simulink library "Regler"  (R2021a)
settings: Solver=ode45  StartTime=0.0  StopTime=10.0  RelTol=1e-3
undefined symbols (not defined in the file or in its folder): k, sfunyst, sync
libraries: $bdroot x3, simulink x1
settings Model: Creator=WL  LastModifiedBy=wll
settings SolverCC: AlgebraicLoopSolver=TrustRegion
settings DataIOCC: LimitDataPoints=on  SaveFormat=Array  SignalLoggingSaveFormat=ModelDataLogs  ReturnWorkspaceOutputs=off
settings OptimizationCC: BooleanDataType=off  ExpressionDepthLimit=2147483647  InitFltsAndDblsToZero=on  LifeSpan=inf
settings DebuggingCC: SaveWithParameterizedLinksMsg=none  UnderspecifiedInitializationDetection=Classic  MergeDetectMultiDrivingBlocksExec=none  SignalResolutionControl=TryResolveAllWithWarning  MultiTaskDSMMsg=warning  MultiTaskCondExecSysMsg=none  FcnCallInpInsideContextMsg=warning  AllowSymbolicDim=off  StateNameClashWarn=warning  SFUnexpectedBacktrackingDiag=warning  SFNoUnconditionalDefaultTransitionDiag=warning  SFExecutionAtInitializationDiag=none  ArithmeticOperatorsInVariantConditions=warning
settings HardwareCC: ProdBitPerPointer=32  ProdBitPerSizeT=32  ProdBitPerPtrDiffT=32  ProdLargestAtomicFloat=None  ProdIntDivRoundTo=Undefined  ProdEndianess=Unspecified  ProdWordSize=32  ProdHWDeviceType=32-bit Generic  TargetUnknown=on
settings ModelReferenceCC: PropagateSignalLabelsOutOfModel=off
settings SFSimCC: SimUseLocalCustomCode=off  CustomCodeUndefinedFunction=UseInterfaceOnly
settings RTWCC: RTWUseLocalCustomCode=off
settings CodeAppCC: StateflowObjectComments=on
settings GRTTargetCC: TargetFcnLib=ansi_tfl_tmw.mat  TargetLangStandard=C89/C90 (ANSI)  CombineOutputUpdateFcns=off  GRTInterface=on
settings ConfigComp: CovMetricSettings=dw  CovSaveCumulativeToWorkspaceVar=on  CovSaveSingleToWorkspaceVar=on  CovExternalEMLEnable=off

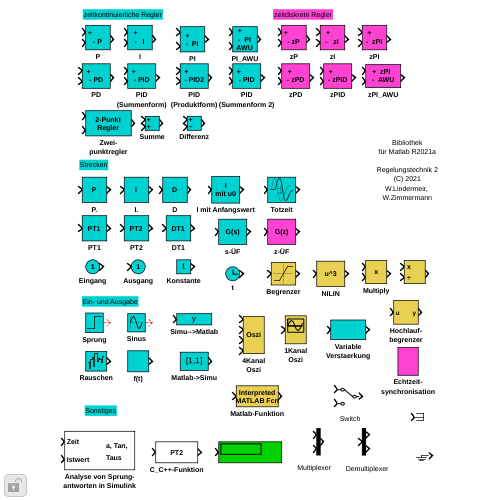
[thumbnail: Simulink's stored preview of the top-level diagram]
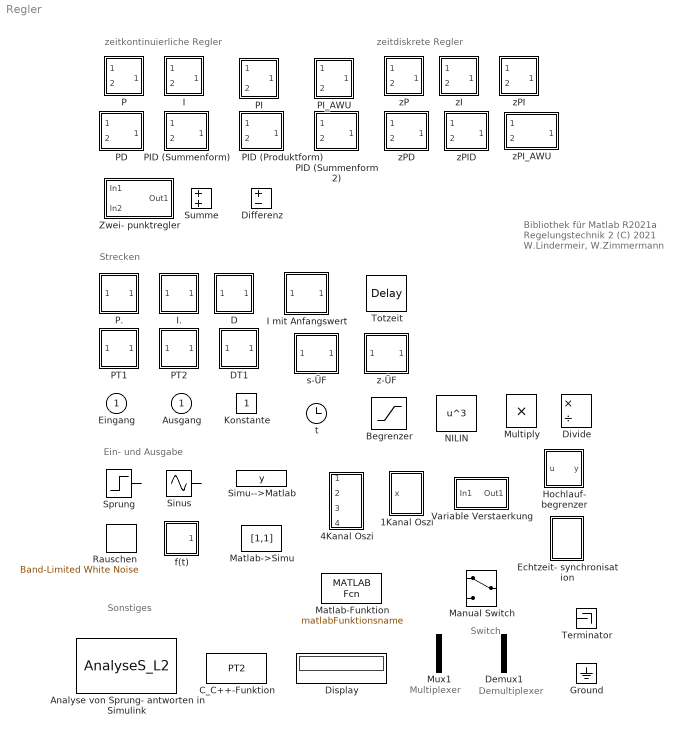
== system Regler ==
  note: Switch
  note: Ein- und Ausgabe
  note: Strecken
  note: zeitdiskrete Regler
  note: zeitkontinuierliche Regler
  note: Bibliothek
      | für Matlab R2021a
      |
      | Regelungstechnik 2
      | (C) 2021
      | W.Lindermeir,
      | W.Zimmermann
  note: Demultiplexer
  note: Multiplexer
  note: Sonstiges
  Eingang : Inport
  1Kanal Oszi : Subsystem  mask(Storage scope.){TR=1, ymin=0, ymax=1, npts=inf, color='r-/b-/g-/m-'}
      mask prompts: TR "Initial Time Range:"; ymin "Initial y-min:"; ymax "Initial y-max:"; npts "Storage pts.:"; color "Line type (rgbw-.:xo):"
      mask help:
      | Storage scope using MATLAB graph window.
      | Enter plotting ranges and line type.
      mask init:
      | ax = [0, TR, ymin, ymax]; dt=-1;
      mask Help: This block uses a MATLAB figure window to plot the input signal.  The graph limits are automatically scaled to the min and max values of the signal stored in the scope's signal buffer.  Line type must be in quotes.  See the M-file sfunyst.m.
      mask Display: plot(0,0,100,100,[83,76,63,52,42,38,28,16,11,84,11,11,11,90,90,11],[75,58,47,54,72,80,84,74,65,65,65,90,40,40,90,90])
  4Kanal Oszi : Subsystem  mask(Oszilloskop){N=20000, k=[1 1 1 1], y=[-5 5], tmax=1}
      mask prompts: N "maximale Anzahl der Abtastpunkte N:"; k "Kanalverstaerkungen:"; y "[ymin ymax]:"
      mask help:
      | 4 Kanal Oszilloskop
      | Kanal1:rot    Kanal2:blau
      | Kanal3:grün Kanal4:magenta
      |
      | Achtung: Wenn das 4 Kanal Oszilloskop mehrfach in einem Blockschaltbild
      | verwendet  wird, müssen die Bezeichnungen der Variablen x1, ..., x4 und t in
      | den Simulink->Matlab Blöcken geändert werden (Edit - Look under Mask),
      | sonst überschreiben die Signale eines Oszilloskops die Werte des anderen
      | Oszilloskops im Matlab-Workspace.
      mask Help: 4 Kanal Oszilloskop mit automat. Skalierung\nKanalverstärkung einstellbar\nKanal1:rot, Kanal2:blau\nKanal3:grün, Kanal4:magenta
      mask Display: disp('Oszi')
  Analyse von Sprung- antworten in Simulink : M-S-Function  FunctionName=AnalyseS_L2  Parameters=tol  mask(Analyse von Sprungantworten){tol=5}
      mask prompts: tol "Toleranzbereich (in %), z.B. +/-5% --> Eingabe 5"
      mask help:
      | Berechnung der Überschwingweite a, der Anregelzeit Tan und der Ausregelzeit Taus.
      |
      | Der Blockeingang ist an den Ausgang der Regelstrecke anzuschliessen.
      |
      | Die Sprungantwort muss am Ende des Zeitbereich eingeschwungen sein. Der Sprung sollte am Anfang des Zeitbereichs erfolgen.
      mask Display:
      | port_label('input',1,'Zeit');
      | port_label('input',2,'Istwert');
      | text(.6,.65,'a, Tan,');
      | text(0.6,.35,'Taus');
  Begrenzer : Saturate
  C_C++-Funktion : S-Function  FunctionName=PT2  Parameters=T  SFunctionDeploymentMode=off  EnableBusSupport=off
  D : Subsystem  mask(D){Td=1}
      mask prompts: Td "Differentiationszeitkonstante Td"
      mask help: D-Glied sTd
      mask Help: D-Glied mit Differentiationszeitkonstante Td
      mask Display: disp('D')
  DT1 : Subsystem  mask(DT1-Glied){Td=5, T1=1}
      mask help: DT1-Glied sTd/(1+sT1)
      mask Help: DT1-Glied
      mask Display: disp('DT1')
  Demux1 : Demux  Outputs=2
  Differenz : Sum  Inputs=+-  InputSameDT=on  SaturateOnIntegerOverflow=on  OutDataTypeStr=Inherit: Same as first input
  Display : Display
  Divide : Product  Inputs=*/
  Echtzeit- synchronisation : Subsystem  mask(Synchronisationsblock){T=0.1}
      mask prompts: T "Synchronistaionsperiode (min. 10ms)"
      mask help:
      | Dieser Block synchronisiert die Simulationszeit mit der realen Zeit, d.h. die Simulation läuft genauso schnell wie die reale Zeit.
      | Die Synchronisation funktioniert nur, wenn der Simulator schneller simuliert als es der realen Zeit entspricht. Der Simulator wird dann jeweils so lange angehalten, bis die reale Zeit wieder "aufgeholt" hat. Der zeitliche Abstand der Wartephasen wird durch den Parameter Synchronisationsperiode T vorgegeben. Falls dieser Block in einem Modell mit zeitdiskreten Blöcken eingesetzt wird, sollte die Synchronisationsperiode auf die (kleinste) Abtastzeit des Modells gesetzt werden. Die Synchronisationsperiode muss >= 10ms sein.
  Ground : Ground
  Hochlauf- begrenzer : Subsystem  mask(Hochlaufbegrenzer){dudt=5}
      mask prompts: dudt "Max. Änderungsgeschwindigkeit (Einheit 1/sec):"
      mask help:
      | Das Ausgangssignal folgt dem zeitlichen Verlauf des Eingangssignals exakt,
      | solange sich das Eingangssignal nicht schneller ändert als +/- du/dt. Wenn
      | sich das Eingangssignal schneller ändert, wird die Änderungsgeschwindigkeit
      | begrenzt.
  I : Subsystem  mask(I){Ti=1}
      mask prompts: Ti "Integrationszeitkonstante Ti"
      mask help: I-Glied 1/sTi
      mask Help: I-Glied mit Integrationszeitkonstante Ti
      mask Display: disp('+    \n-   I')
  I mit Anfangswert : Subsystem  mask(I-Glied 1/sTi mit Anfangswert u0){Ti=1100, u0=60}
      mask prompts: Ti "Integrationszeitkonstante Ti"; u0 "Anfangswert"
      mask help: I-Glied mit Anfangswert u0
      mask Help: Integralglied mit Anfangswert zum Zeitpunkt 0
      mask Display: disp('I\nmit u0')
  I. : Subsystem  mask(I){Ti=1}
      mask prompts: Ti "Integrationszeitkonstante Ti"
      mask help: I-Glied 1/sTi
      mask Help: I-Glied mit Integrationszeitkonstante Ti
      mask Display: disp('I')
  Konstante : Constant
  Manual Switch : ManualSwitch
  Matlab->Simu : FromWorkspace  VariableName=[1,1]  SampleTime=-1  ZeroCross=off
  Matlab-Funktion : MATLABFcn  MATLABFcn=matlabFunktionsname  OutputDimensions=3  Output1D=off
  Multiply : Product  Inputs=**
  Mux1 : Mux  Inputs=2
  NILIN : Fcn  Expr=u^3
  P : Subsystem  mask(P-Regler){kp=1}
      mask help: P
      mask Help: P-Regler mit Proportionalfaktor kp
      mask Display: disp('+        \n- P')
  P. : Subsystem  mask(P){k=1}
      mask prompts: k "Verstärkung k"
      mask help: P-Glied k
      mask Help: P-Glied mit Verstärkung k
      mask Display: disp('P')
  PD : Subsystem  mask(PD-Regler){kp=1, Tv=1, T1=0}
      mask help: PD(T1) kp (1+sTv) / (1+sT1)
      mask Help:
      | PD-Regler mit Proportionalfaktor kp und Differentiationszeitkonstante Tv.
      | Der D-Anteil wird durch ein DT1-Glied mit der zusätzlichen Tiefpasszeitkonstante T1 angenähert, es muss sein T1 >= Tv/100.
      mask Display: disp('+        \n- PD')
  PI : Subsystem  mask(PI){kp=1, Tn=1}
      mask help: PI-Regler kp (1+1/sTn)
      mask Help: PI-Regler mit Verstärkung kp und Nachstellzeit Tn
      mask Display: disp('+     \n-  PI')
  PID (Produktform) : Subsystem  mask(PID-Regler in Produktform){kr=1, Ti=1, Td=0.1, T1=0}
      mask prompts: T1 "T1  -- Achtung: Intern T1 = max(Td/100,T1)"
      mask help: PID(T1) in Produktform kr (1+sTi) (1+sTd) / sTi (1+sT1)
      mask Help:
      | PID-Regler in Produktform mit Proportionalfaktor kr, Integrationszeitkonstante Ti und Differentiationszeitkonstante Td.
      | Der D-Anteil wird durch ein DT1-Glied mit der zusätzlichen Tiefpasszeitkonstante T1 angenähert, es muss sein T1 >= Td/100.
      mask Display: disp('+        \n- PID2')
  PID (Summenform 2) : Subsystem  mask(PID-Regler in Summenform){kp=1, ki=0, kv=0, T1=0}
      mask help: PID(T1) in alternativer Summenform kp + ki/s + skv/(1+sT1) )
      mask Help:
      | PID-Regler in Summenform mit Proportionalverstärkung kp, Integralverstärkung ki und Differentialverstärkung kv.
      | Der D-Anteil wird durch ein DT1-Glied mit der zusätzlichen Tiefpasszeitkonstante T1 angenähert.
      mask Display: disp('+        \n- PID')
  PID (Summenform) : Subsystem  mask(PID-Regler in Summenform){kp=1, Tn=1, Tv=0.1, T1=0}
      mask prompts: T1 "T1  -- Achtung: Intern T1 = max(Tv/100,T1)"
      mask help: PID(T1) in Summenform kp ( 1+ 1/sTn + sTv/(1+sT1) )
      mask Help:
      | PID-Regler in Summenform mit Proportionalfaktor kp, Integrationszeitkonstante Tn (Nachstellzeit) und Differentiationszeitkonstante Tv (Vorhaltezeit).
      | Der D-Anteil wird durch ein DT1-Glied mit der zusätzlichen Tiefpasszeitkonstante T1 angenähert, es muss sein T1 >= Tv/100.
      mask Display: disp('+        \n- PID')
  PI_AWU : Subsystem  AncestorBlock=Regler/PI  mask(PI-Regler mit Anti-Windup){kp=1, Tn=0.01, bo=inf, bu=-inf}
      mask prompts: bo "Obere Begrenzung:"; bu "Untere Begrenzung:"
      mask help: PI mit Anti-Windup kp (1+sTn) / sTn
      mask Help: PI-Regler mit Proportionalfaktor kP und Integrationszeitkonstante Tn. Das Ausgangssignal wird auf den Bereich bu ... bo begrenzt. Das Einschwingverhalten bei Begrenzung wird durch eine Anti-Windup-Massnahme verbessert.
      mask Display: disp('+     \n-  PI\nAWU')
  PT1 : Subsystem  mask(PT1){k=1, T1=1}
      mask prompts: k "Verstärkung kp"; T1 "Zeitkonstante T1"
      mask help: PT1-Glied kp/(1+s·T1)
      mask Help: PT1 Tiefpaß 1.Ordnung mit Verstärkung kp und Zeitkonstante T1
      mask Display: disp('PT1')
  PT2 : Subsystem  mask(PT2){k=1, T=1, D=1}
      mask prompts: k "Verstärkung kp"; T "Zeitkonstante T1"; D "Dämpfung D"
      mask help: PT2-Glied kp/(1+s·2D·T1+s²T1²)
      mask Help: PT2 Tiefpaß 2.Ordnung mit Verstärkung kp, Zeitkonstante T1 und Daempfung D
      mask Display: disp('PT2')
  Rauschen : simulink/Sources/Band-Limited White Noise  Cov=[0.1]  Ts=0.1  seed=[23341]
  Simu-->Matlab : ToWorkspace  VariableName=y
      settings: MaxDataPoints=10000
  Sinus : Sin
  Sprung : Step  Time=0.000001  SampleTime=0
  Summe : Sum  InputSameDT=on  SaturateOnIntegerOverflow=on  OutDataTypeStr=Inherit: Same as first input
  Terminator : Terminator
  Totzeit : TransportDelay
  Variable Verstaerkung : Subsystem  LoadFcn=slideg Load  mask{Parameter4=40, k=k, Parameter5=160}
      mask prompts: Parameter4 "Low"; k "Gain"; Parameter5 "High"
      settings: CopyFcn=slideg Copy  DeleteFcn=slideg DeleteBlock  NameChangeFcn=slideg NameChange  OpenFcn=slideg Open  ParentCloseFcn=slideg ParentClose
      mask Display: disp(k)
  Zwei- punktregler : Subsystem  mask(Zweipunktregler){Yo=1, Yu=-1, So=0.1, Su=-0.1}
      mask prompts: Yo "Ausgangsignal oberer Wert:"; Yu "Ausgangssignal unterer Wert:"; So "Schaltschwelle oberer Wert:"; Su "Schaltschwelle unterer Wert:"
      mask help: Zweipunktregler mit Hysterese
      mask Help: Zweipunktregler mit Hysterese
      mask Display: fprintf('2-Punkt\nRegler')
  f(t) : Subsystem
  s-ÜF : Subsystem  mask(G(s)){Z=[0 1], N=[1 1]}
      mask prompts: Z "Zähler:"; N "Nenner:"
      mask help: zeitkontinuierliche Uebertragungsfunktion
      mask Help: beliebige Uebertragungsfunktion G(s)=Z(s)/N(s)
      mask Display: disp('G(s)')
  t : Clock
  z-ÜF : Subsystem  mask(beliebige z-Übertragungsfunktion){Z=[0 1], N=[1 1], T=1}
      mask prompts: Z "Zähler:"; N "Nenner:"; T "Abtastzeit T:"
      mask help: beliebige z-Übertragungsfunktion G(z)
      mask Help: beliebige z-Übertragungsfunktion\nG(s)=Z(z)/N(z)
      mask Display: disp('G(z)')
  zI : Subsystem  mask(zI){Ti=1, T=1}
      mask prompts: Ti "Integrationszeitkonstante Ti"; T "Abtastzeit T"
      mask help: zeitdiskreter I-Regler T/Ti z/z-1
      mask Help: zeitdiskretesI-Glied mit Integrationszeitkonstante Ti und Abtastzeit T
      mask Display: disp('+    \n-   zI')
  zP : Subsystem  mask(zP){kp=1, T=1}
      mask prompts: T "Abtastzeit T"
      mask help: P
      mask Help: zeitdiskreter P-Regler mit Proportionalfaktor kp und Abtastzeit T
      mask Display: disp('+        \n- zP')
  zPD : Subsystem  mask(zPD){kp=1, Td=1, T=1}
      mask help: zeitdiskreter PD-Regler kp (1+Td/T (z-1)/z)
      mask Help: zeitdiskreter PD-Regler mit Verstärkung kp, Differentiationszeitkonstante Td und Abtastzeit T
      mask Display: disp('+      \n- zPD')
  zPI : Subsystem  mask(zPI){kp=1, Tn=1, T=1}
      mask prompts: T "Abtastzeit T"
      mask help: zeitdiskreter PI-Regler kp (1+T/Tn z/z-1)
      mask Help: zeitdiskreter PI-Regler mit Verstärkung kp, Nachstellzeit Tn und Abtastzeit T
      mask Display: disp('+     \n-  zPI')
  zPID : Subsystem  mask(zPID in Normalform){kp=1, Tn=1, Tv=1, T=1}
      mask help: zeitdiskreter PID-Regler (Normalform) kp (1+T/Tn z/z-1+Tv/T (z-1)/z)
      mask Help: zeitdiskreter PID-Regler in Normalform mit Verstärkung kp, Nachstellzeit Tn, Vorhaltezeit Tv und Abtastzeit T
      mask Display: disp('+       \n- zPID')
  zPI_AWU : Subsystem  mask(zPI_AWU){kp=1, Tn=1, T=1, bo=inf, bu=-inf}
      mask prompts: T "Abtastzeit T:"; bo "obere Begrenzung bo:"; bu "untere Begrenzung bu:"
      mask help: zeitdiskreter PI-Regler kp (1+T/Tn z/z-1) mit Anti-Windup-Begrenzung
      mask Help: zeitdiskreter Anti-Windup-PI-Regler\nmit Verstärkung kp, Nachstellzeit Tn\nund Abtastzeit T,\nobere und untere Begrenzung bu, bo.\nAls Anti-Windup-Massnahme wird der Integralanteil angehalten, wenn der Reglerausgang in die Begrenzung geht.
      mask Display: disp('+  zPI  \n-  AWU')
  Ausgang : Outport  VectorParamsAs1DForOutWhenUnconnected=off
  wires:
  Sinus/1 -> ?
  Sprung/1 -> ?

== system Regler/1Kanal Oszi ==
  x : Inport
  "S-function M-file which plots lines " : S-Function  LoadFcn=sfunyst([],[],[],'LoadBlock')  FunctionName=sfunyst  Parameters=ax, color, npts, dt  SFunctionDeploymentMode=off  EnableBusSupport=off
      settings: CopyFcn=sfunyst([],[],[],'CopyBlock')  DeleteFcn=sfunyst([],[],[],'DeleteBlock')
  wires:
  x/1 -> "S-function M-file which plots lines "/1

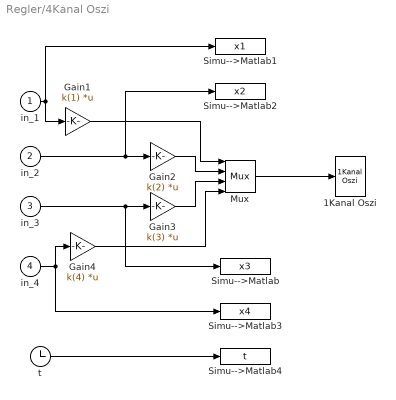
== system Regler/4Kanal Oszi ==
  in_1 : Inport
  in_2 : Inport  Port=2
  in_3 : Inport  Port=3
  in_4 : Inport  Port=4
  1Kanal Oszi : $bdroot/1Kanal Oszi  TR=1  ymin=0  ymax=1  npts=inf  color='r-/b-/g-/m-'
  Gain1 : Gain  Gain=k(1)  Multiplication=Matrix(K*u)  SaturateOnIntegerOverflow=on  OutDataTypeStr=Inherit: Same as input  ParamDataTypeStr=Inherit: Same as input
  Gain2 : Gain  Gain=k(2)  Multiplication=Matrix(K*u)  SaturateOnIntegerOverflow=on  OutDataTypeStr=Inherit: Same as input  ParamDataTypeStr=Inherit: Same as input
  Gain3 : Gain  Gain=k(3)  Multiplication=Matrix(K*u)  SaturateOnIntegerOverflow=on  OutDataTypeStr=Inherit: Same as input  ParamDataTypeStr=Inherit: Same as input
  Gain4 : Gain  Gain=k(4)  Multiplication=Matrix(K*u)  SaturateOnIntegerOverflow=on  OutDataTypeStr=Inherit: Same as input  ParamDataTypeStr=Inherit: Same as input
  Mux : Mux
  Simu-->Matlab : ToWorkspace  VariableName=x3
      settings: MaxDataPoints=N
  Simu-->Matlab1 : ToWorkspace  VariableName=x1
      settings: MaxDataPoints=N
  Simu-->Matlab2 : ToWorkspace  VariableName=x2
      settings: MaxDataPoints=N
  Simu-->Matlab3 : ToWorkspace  VariableName=x4
      settings: MaxDataPoints=N
  Simu-->Matlab4 : ToWorkspace  VariableName=t
      settings: MaxDataPoints=N
  t : Clock
  wires:
  in_1/1 -> Gain1/1, Simu-->Matlab1/1
  Gain1/1 -> Mux/1
  Gain4/1 -> Mux/4
  in_4/1 -> Simu-->Matlab3/1, Gain4/1
  Gain3/1 -> Mux/3
  Gain2/1 -> Mux/2
  in_3/1 -> Gain3/1, Simu-->Matlab/1
  in_2/1 -> Gain2/1, Simu-->Matlab2/1
  Mux/1 -> 1Kanal Oszi/1
  t/1 -> Simu-->Matlab4/1

== system Regler/D ==
  In1 : Inport
  D : TransferFcn  Numerator=[Td]  Denominator=[1]
  Out1 : Outport  VectorParamsAs1DForOutWhenUnconnected=off
  wires:
  D/1 -> Out1/1
  In1/1 -> D/1

== system Regler/DT1 ==
  In1 : Inport
  DT1 : TransferFcn  Numerator="[Td  0]"  Denominator="[T1  1]"
  Out1 : Outport  VectorParamsAs1DForOutWhenUnconnected=off
  wires:
  DT1/1 -> Out1/1
  In1/1 -> DT1/1

== system Regler/Echtzeit- synchronisation ==
  Pause : MATLABFcn  MATLABFcn=sync(u)  OutputDimensions=0  Output1D=off  SampleTime=T
  t : Clock
  wires:
  t/1 -> Pause/1

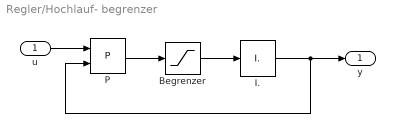
== system Regler/Hochlauf- begrenzer ==
  u : Inport
  Begrenzer : Saturate  UpperLimit=dudt  LowerLimit=-dudt
  I. : $bdroot/I.  Ti=1
  P : $bdroot/P  kp=1
  y : Outport  VectorParamsAs1DForOutWhenUnconnected=off
  wires:
  u/1 -> P/1
  I./1 -> y/1, P/2
  Begrenzer/1 -> I./1
  P/1 -> Begrenzer/1

== system Regler/I ==
  in_1 : Inport
  in_2 : Inport  Port=2
  Differenz1 : Sum  Inputs=+-  InputSameDT=on  SaturateOnIntegerOverflow=on  OutDataTypeStr=Inherit: Same as first input
  I1 : TransferFcn  Denominator="[Ti  0]"
  out_1 : Outport  VectorParamsAs1DForOutWhenUnconnected=off
  wires:
  in_2/1 -> Differenz1/2
  I1/1 -> out_1/1
  in_1/1 -> Differenz1/1
  Differenz1/1 -> I1/1

== system Regler/I mit Anfangswert ==
  Eingang : Inport
  "1_Ti " : Gain  Gain=1/Ti  SaturateOnIntegerOverflow=on  OutDataTypeStr=Inherit: Same as input  ParamDataTypeStr=Inherit: Same as input
  Integrator mit Anfangswert : Integrator  InitialCondition=u0
  Ausgang : Outport  VectorParamsAs1DForOutWhenUnconnected=off
  wires:
  "1_Ti "/1 -> Integrator mit Anfangswert/1
  Eingang/1 -> "1_Ti "/1
  Integrator mit Anfangswert/1 -> Ausgang/1

== system Regler/I. ==
  In1 : Inport
  I. : TransferFcn  Denominator="[Ti  0]"
  Out1 : Outport  VectorParamsAs1DForOutWhenUnconnected=off
  wires:
  I./1 -> Out1/1
  In1/1 -> I./1

== system Regler/P ==
  in_1 : Inport
  in_2 : Inport  Port=2
  Differenz : Sum  Inputs=+-  InputSameDT=on  SaturateOnIntegerOverflow=on  OutDataTypeStr=Inherit: Same as first input
  P : TransferFcn  Numerator=[kp]  Denominator=[1]
  out_1 : Outport  VectorParamsAs1DForOutWhenUnconnected=off
  wires:
  Differenz/1 -> P/1
  P/1 -> out_1/1
  in_1/1 -> Differenz/1
  in_2/1 -> Differenz/2

== system Regler/P. ==
  In1 : Inport
  P. : TransferFcn  Numerator=[k]  Denominator=[1]
  Out1 : Outport  VectorParamsAs1DForOutWhenUnconnected=off
  wires:
  P./1 -> Out1/1
  In1/1 -> P./1

== system Regler/PD ==
  Regel- differenz1 : Inport
  Regel- differenz : Inport  Port=2
  Differenz : Sum  Inputs=+-  InputSameDT=on  SaturateOnIntegerOverflow=on  OutDataTypeStr=Inherit: Same as first input
  PDT1 : TransferFcn  Numerator="[kp*Tv                kp]"  Denominator="[max(Tv/100,T1)   1]"
  Stellgröße : Outport  VectorParamsAs1DForOutWhenUnconnected=off
  wires:
  PDT1/1 -> Stellgröße/1
  Differenz/1 -> PDT1/1
  Regel- differenz/1 -> Differenz/2
  Regel- differenz1/1 -> Differenz/1

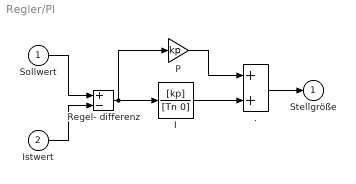
== system Regler/PI ==
  Sollwert : Inport
  Istwert : Inport  Port=2
  . : Sum  InputSameDT=on  SaturateOnIntegerOverflow=on  OutDataTypeStr=Inherit: Same as first input
  I : TransferFcn  Numerator=[kp]  Denominator=[Tn 0]
  P : Gain  Gain=kp  SaturateOnIntegerOverflow=on  OutDataTypeStr=Inherit: Same as input  ParamDataTypeStr=Inherit: Same as input
  Regel- differenz : Sum  Inputs=+-  InputSameDT=on  SaturateOnIntegerOverflow=on  OutDataTypeStr=Inherit: Same as first input
  Stellgröße : Outport  VectorParamsAs1DForOutWhenUnconnected=off
  wires:
  Istwert/1 -> Regel- differenz/2
  Sollwert/1 -> Regel- differenz/1
  ./1 -> Stellgröße/1
  Regel- differenz/1 -> P/1, I/1
  I/1 -> ./2
  P/1 -> ./1

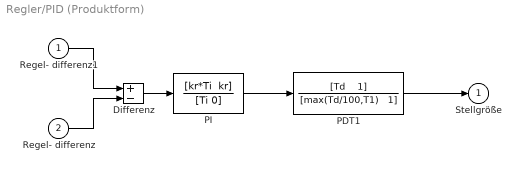
== system Regler/PID (Produktform) ==
  Regel- differenz1 : Inport
  Regel- differenz : Inport  Port=2
  Differenz : Sum  Inputs=+-  InputSameDT=on  SaturateOnIntegerOverflow=on  OutDataTypeStr=Inherit: Same as first input
  PDT1 : TransferFcn  Numerator="[Td    1]"  Denominator="[max(Td/100,T1)   1]"
  PI : TransferFcn  Numerator="[kr*Ti  kr]"  Denominator=[Ti 0]
  Stellgröße : Outport  VectorParamsAs1DForOutWhenUnconnected=off
  wires:
  Regel- differenz1/1 -> Differenz/1
  Regel- differenz/1 -> Differenz/2
  Differenz/1 -> PI/1
  PI/1 -> PDT1/1
  PDT1/1 -> Stellgröße/1

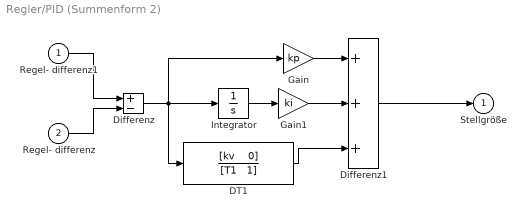
== system Regler/PID (Summenform 2) ==
  Regel- differenz1 : Inport
  Regel- differenz : Inport  Port=2
  DT1 : TransferFcn  Numerator="[kv    0]"  Denominator="[T1   1]"
  Differenz : Sum  Inputs=+-  InputSameDT=on  SaturateOnIntegerOverflow=on  OutDataTypeStr=Inherit: Same as first input
  Differenz1 : Sum  Inputs=+++  InputSameDT=on  SaturateOnIntegerOverflow=on  OutDataTypeStr=Inherit: Same as first input
  Gain : Gain  Gain=kp
  Gain1 : Gain  Gain=ki
  Integrator : Integrator
  Stellgröße : Outport  VectorParamsAs1DForOutWhenUnconnected=off
  wires:
  Integrator/1 -> Gain1/1
  Gain1/1 -> Differenz1/2
  Differenz1/1 -> Stellgröße/1
  Differenz/1 -> Integrator/1, Gain/1, DT1/1
  DT1/1 -> Differenz1/3
  Gain/1 -> Differenz1/1
  Regel- differenz/1 -> Differenz/2
  Regel- differenz1/1 -> Differenz/1

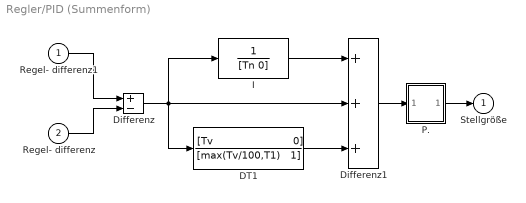
== system Regler/PID (Summenform) ==
  Regel- differenz1 : Inport
  Regel- differenz : Inport  Port=2
  DT1 : TransferFcn  Numerator="[Tv                        0]"  Denominator="[max(Tv/100,T1)   1]"
  Differenz : Sum  Inputs=+-  InputSameDT=on  SaturateOnIntegerOverflow=on  OutDataTypeStr=Inherit: Same as first input
  Differenz1 : Sum  Inputs=+++  InputSameDT=on  SaturateOnIntegerOverflow=on  OutDataTypeStr=Inherit: Same as first input
  I : TransferFcn  Denominator=[Tn 0]
  P. : Subsystem  mask(P){k=kp}
      mask prompts: k "Verstärkung k"
      mask help: P-Glied k
      mask Help: P-Glied mit Verstärkung k
      mask Display: disp('P')
  Stellgröße : Outport  VectorParamsAs1DForOutWhenUnconnected=off
  wires:
  Differenz1/1 -> P./1(In1)
  P./1(Out1) -> Stellgröße/1
  Differenz/1 -> Differenz1/2, I/1, DT1/1
  DT1/1 -> Differenz1/3
  I/1 -> Differenz1/1
  Regel- differenz/1 -> Differenz/2
  Regel- differenz1/1 -> Differenz/1

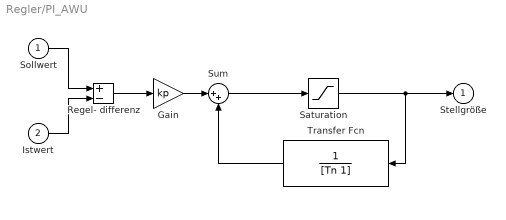
== system Regler/PI_AWU ==
  Sollwert : Inport
  Istwert : Inport  Port=2
  Gain : Gain  Gain=kp
  Regel- differenz : Sum  Inputs=+-  InputSameDT=on  SaturateOnIntegerOverflow=on  OutDataTypeStr=Inherit: Same as first input
  Saturation : Saturate  UpperLimit=bo  LowerLimit=bu
  Sum : Sum  Inputs=|++
  Transfer Fcn : TransferFcn  Denominator=[Tn 1]
  Stellgröße : Outport  VectorParamsAs1DForOutWhenUnconnected=off
  wires:
  Istwert/1 -> Regel- differenz/2
  Sollwert/1 -> Regel- differenz/1
  Regel- differenz/1 -> Gain/1
  Gain/1 -> Sum/1
  Sum/1 -> Saturation/1
  Saturation/1 -> Transfer Fcn/1, Stellgröße/1
  Transfer Fcn/1 -> Sum/2

== system Regler/PT1 ==
  In1 : Inport
  PT1 : TransferFcn  Numerator=[k]  Denominator="[T1  1]"
  Out1 : Outport  VectorParamsAs1DForOutWhenUnconnected=off
  wires:
  PT1/1 -> Out1/1
  In1/1 -> PT1/1

== system Regler/PT2 ==
  In1 : Inport
  PT2 : TransferFcn  Numerator=[k]  Denominator="[T^2  2*D*T  1]"
  Out1 : Outport  VectorParamsAs1DForOutWhenUnconnected=off
  wires:
  PT2/1 -> Out1/1
  In1/1 -> PT2/1

== system Regler/Variable Verstaerkung ==
  In1 : Inport
  Variable Verstaerkung : Gain  Gain=k  SaturateOnIntegerOverflow=on  OutDataTypeStr=Inherit: Same as input  ParamDataTypeStr=Inherit: Same as input
  Out1 : Outport  VectorParamsAs1DForOutWhenUnconnected=off
  wires:
  Variable Verstaerkung/1 -> Out1/1
  In1/1 -> Variable Verstaerkung/1

== system Regler/Zwei- punktregler ==
  In1 : Inport
  In2 : Inport  Port=2
  Differenz : Sum  Inputs=+-  InputSameDT=on  SaturateOnIntegerOverflow=on  OutDataTypeStr=Inherit: Same as first input
  Zwei- punktregler : Relay  OnSwitchValue=So  OffSwitchValue=Su  OnOutputValue=Yo  OffOutputValue=Yu
  Out1 : Outport  VectorParamsAs1DForOutWhenUnconnected=off
  wires:
  In2/1 -> Differenz/2
  In1/1 -> Differenz/1
  Differenz/1 -> Zwei- punktregler/1
  Zwei- punktregler/1 -> Out1/1

== system Regler/f(t) ==
  f(t) : Fcn  Expr=sin(u)
  t : Clock
  out_1 : Outport  VectorParamsAs1DForOutWhenUnconnected=off
  wires:
  f(t)/1 -> out_1/1
  t/1 -> f(t)/1

== system Regler/s-ÜF ==
  In1 : Inport
  s-ÜF : TransferFcn  Numerator=Z  Denominator=N
  Out1 : Outport  VectorParamsAs1DForOutWhenUnconnected=off
  wires:
  s-ÜF/1 -> Out1/1
  In1/1 -> s-ÜF/1

== system Regler/z-ÜF ==
  In1 : Inport
  z-ÜF : DiscreteTransferFcn  Numerator=Z  Denominator=N  SampleTime=T
  Out1 : Outport  VectorParamsAs1DForOutWhenUnconnected=off
  wires:
  z-ÜF/1 -> Out1/1
  In1/1 -> z-ÜF/1

== system Regler/zI ==
  in_1 : Inport
  in_2 : Inport  Port=2
  Differenz1 : Sum  Inputs=+-  InputSameDT=on  SaturateOnIntegerOverflow=on  OutDataTypeStr=Inherit: Same as first input
  Discrete Transfer Fcn : DiscreteTransferFcn  Numerator=[T/Ti 0]  Denominator=[1 -1]  SampleTime=T
  out_1 : Outport  VectorParamsAs1DForOutWhenUnconnected=off
  wires:
  Differenz1/1 -> Discrete Transfer Fcn/1
  in_1/1 -> Differenz1/1
  Discrete Transfer Fcn/1 -> out_1/1
  in_2/1 -> Differenz1/2

== system Regler/zP ==
  sollwert : Inport
  istwert : Inport  Port=2
  Differenz : Sum  Inputs=+-  InputSameDT=on  SaturateOnIntegerOverflow=on  OutDataTypeStr=Inherit: Same as first input
  P : DiscreteTransferFcn  Numerator=[kp]  Denominator=[1]  SampleTime=T
  stellgroesse : Outport  VectorParamsAs1DForOutWhenUnconnected=off
  wires:
  istwert/1 -> Differenz/2
  sollwert/1 -> Differenz/1
  P/1 -> stellgroesse/1
  Differenz/1 -> P/1

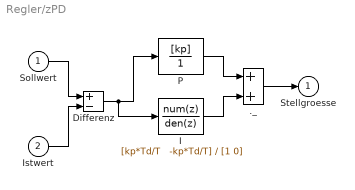
== system Regler/zPD ==
  Sollwert : Inport
  Istwert : Inport  Port=2
  ._ : Sum  InputSameDT=on  SaturateOnIntegerOverflow=on  OutDataTypeStr=Inherit: Same as first input
  Differenz : Sum  Inputs=+-  InputSameDT=on  SaturateOnIntegerOverflow=on  OutDataTypeStr=Inherit: Same as first input
  I : DiscreteTransferFcn  Numerator="[kp*Td/T   -kp*Td/T]"  Denominator=[1 0]  SampleTime=T
  P : DiscreteTransferFcn  Numerator=[kp]  Denominator=[1]  SampleTime=T
  Stellgroesse : Outport  VectorParamsAs1DForOutWhenUnconnected=off
  wires:
  I/1 -> ._/2
  ._/1 -> Stellgroesse/1
  P/1 -> ._/1
  ? -> ?
  Differenz/1 -> I/1, P/1
  Sollwert/1 -> Differenz/1
  Istwert/1 -> Differenz/2

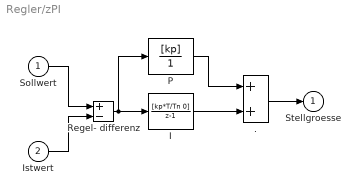
== system Regler/zPI ==
  Sollwert : Inport
  Istwert : Inport  Port=2
  . : Sum  InputSameDT=on  SaturateOnIntegerOverflow=on  OutDataTypeStr=Inherit: Same as first input
  I : DiscreteTransferFcn  Numerator=[kp*T/Tn 0]  Denominator=[1 -1]  SampleTime=T
  P : DiscreteTransferFcn  Numerator=[kp]  Denominator=[1]  SampleTime=T
  Regel- differenz : Sum  Inputs=+-  InputSameDT=on  SaturateOnIntegerOverflow=on  OutDataTypeStr=Inherit: Same as first input
  Stellgroesse : Outport  VectorParamsAs1DForOutWhenUnconnected=off
  wires:
  P/1 -> ./1
  I/1 -> ./2
  Regel- differenz/1 -> I/1, P/1
  ./1 -> Stellgroesse/1
  Sollwert/1 -> Regel- differenz/1
  Istwert/1 -> Regel- differenz/2

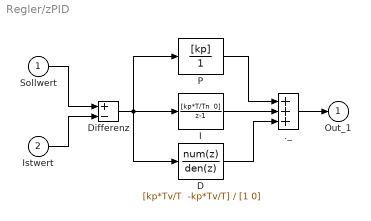
== system Regler/zPID ==
  Sollwert : Inport
  Istwert : Inport  Port=2
  ._ : Sum  Inputs=+++  InputSameDT=on  SaturateOnIntegerOverflow=on  OutDataTypeStr=Inherit: Same as first input
  D : DiscreteTransferFcn  Numerator="[kp*Tv/T  -kp*Tv/T]"  Denominator=[1 0]  SampleTime=T
  Differenz : Sum  Inputs=+-  InputSameDT=on  SaturateOnIntegerOverflow=on  OutDataTypeStr=Inherit: Same as first input
  I : DiscreteTransferFcn  Numerator="[kp*T/Tn  0]"  Denominator=[1 -1]  SampleTime=T
  P : DiscreteTransferFcn  Numerator=[kp]  Denominator=[1]  SampleTime=T
  Out_1 : Outport  VectorParamsAs1DForOutWhenUnconnected=off
  wires:
  ._/1 -> Out_1/1
  D/1 -> ._/3
  I/1 -> ._/2
  P/1 -> ._/1
  Sollwert/1 -> Differenz/1
  Istwert/1 -> Differenz/2
  Differenz/1 -> P/1, D/1, I/1

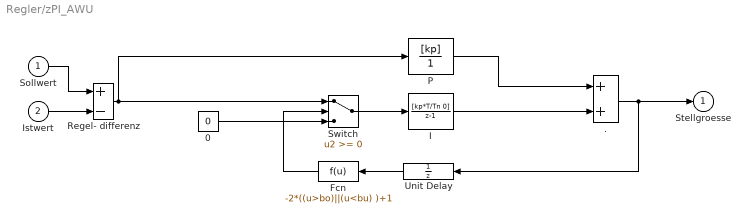
== system Regler/zPI_AWU ==
  Sollwert : Inport
  Istwert : Inport  Port=2
  . : Sum  InputSameDT=on  SaturateOnIntegerOverflow=on  OutDataTypeStr=Inherit: Same as first input
  0 : Constant  Value=0
  Fcn : Fcn  Expr=-2*((u>bo)||(u<bu) )+1
  I : DiscreteTransferFcn  Numerator=[kp*T/Tn 0]  Denominator=[1 -1]  SampleTime=T
  P : DiscreteTransferFcn  Numerator=[kp]  Denominator=[1]  SampleTime=T
  Regel- differenz : Sum  Inputs=+-  InputSameDT=on  SaturateOnIntegerOverflow=on  OutDataTypeStr=Inherit: Same as first input
  Switch : Switch  SaturateOnIntegerOverflow=on  InputSameDT=on
  Unit Delay : UnitDelay  SampleTime=T  HasFrameUpgradeWarning=on
  Stellgroesse : Outport  VectorParamsAs1DForOutWhenUnconnected=off
  wires:
  I/1 -> ./2
  Regel- differenz/1 -> P/1, Switch/1
  Istwert/1 -> Regel- differenz/2
  P/1 -> ./1
  Switch/1 -> I/1
  0/1 -> Switch/3
  Sollwert/1 -> Regel- differenz/1
  ./1 -> Unit Delay/1, Stellgroesse/1
  Unit Delay/1 -> Fcn/1
  Fcn/1 -> Switch/2

== system Regler/PID (Summenform)/P. ==
  In1 : Inport
  P. : TransferFcn  Numerator=[k]  Denominator=[1]
  Out1 : Outport  VectorParamsAs1DForOutWhenUnconnected=off
  wires:
  P./1 -> Out1/1
  In1/1 -> P./1
